simulink model "wheel_robot"  (R2019b)
settings: Solver=ode4  StartTime=0.0  StopTime=33  FixedStep=1e-2  RelTol=1e-3
values from neighbouring files (symbols this model uses):
  dt = 1e-2    (= 0.01)    [init.m]
  g = [0 0 -10]    [init.m]
  gps_pos_local_rsm = 1.66    [init.m]
  gps_vel_local_rsm = 0.05    [init.m]
  imu_acc_rsm = 0.25    [init.m]
  imu_rot_vel_rsm = 0.05    [init.m]
  initial_ctrl = [0;0]    [init.m]
  initial_state_local = [0;0;0]    [init.m]
  sqrtP0 = chol(P0,'lower')    [init.m]
  sqrtQ = chol(Q,'lower')    [init.m]
  sqrtR = chol(R,'lower')    [init.m]
  X0 = [0 0 0    0 0 0    0 0 0]'    [init.m]
libraries: simulink x1
settings Model: Creator=shawinmihail  LastModifiedBy=shawinmihail

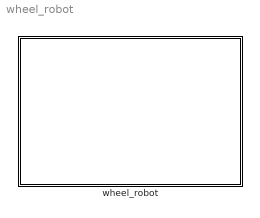
== system wheel_robot ==
  wheel_robot : Subsystem  InitFcn=init

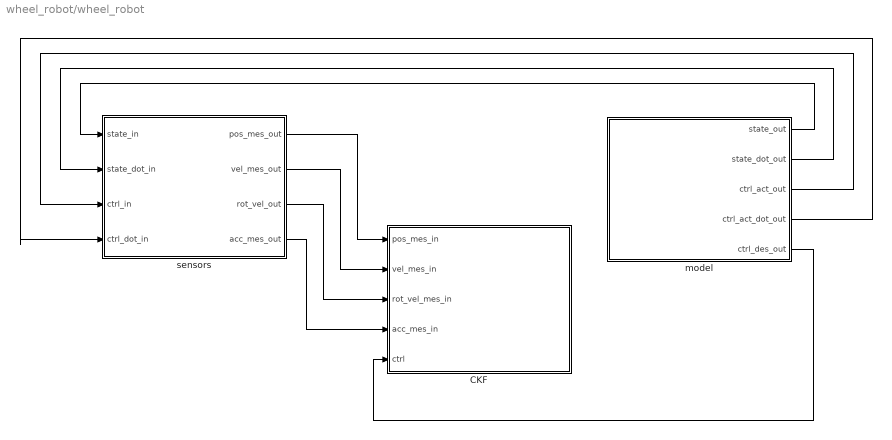
== system wheel_robot/wheel_robot ==
  CKF : Subsystem  InitFcn=init
  model : Subsystem
  sensors : Subsystem  InitFcn=init
  wires:
  model/2(state_dot_out) -> sensors/2(state_dot_in)
  model/1(state_out) -> sensors/1(state_in)
  model/3(ctrl_act_out) -> sensors/3(ctrl_in)
  model/4(ctrl_act_dot_out) -> sensors/4(ctrl_dot_in)
  sensors/4(acc_mes_out) -> CKF/4(acc_mes_in)
  sensors/3(rot_vel_out) -> CKF/3(rot_vel_mes_in)
  sensors/2(vel_mes_out) -> CKF/2(vel_mes_in)
  sensors/1(pos_mes_out) -> CKF/1(pos_mes_in)
  model/5(ctrl_des_out) -> CKF/5(ctrl)

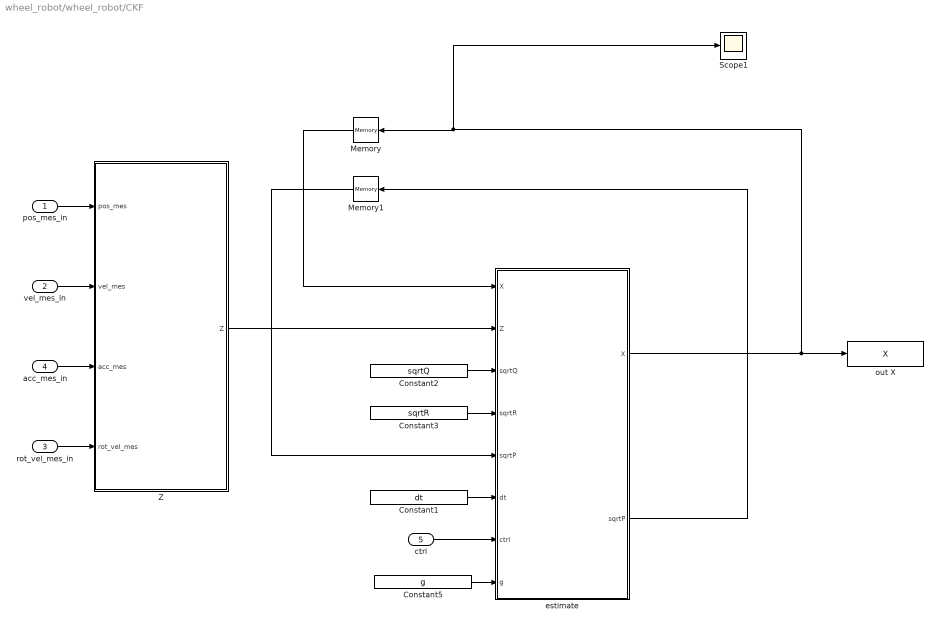
== system wheel_robot/wheel_robot/CKF ==
  pos_mes_in : Inport
  vel_mes_in : Inport  Port=2
  rot_vel_mes_in : Inport  Port=3
  acc_mes_in : Inport  Port=4
  ctrl : Inport  Port=5
  Constant1 : Constant  Value=dt
  Constant2 : Constant  Value=sqrtQ
  Constant3 : Constant  Value=sqrtR
  Constant5 : Constant  Value=g
  Memory : Memory  InitialCondition=X0
  Memory1 : Memory  InitialCondition=sqrtP0
  Scope1 : Scope
  Z : MATLAB Function  TreatAsAtomicUnit=on
  estimate : MATLAB Function  TreatAsAtomicUnit=on
  out X : ToWorkspace  VariableName=X  SaveFormat=Timeseries  SampleTime=-1
  wires:
  pos_mes_in/1 -> Z/1(pos_mes)
  vel_mes_in/1 -> Z/2(vel_mes)
  acc_mes_in/1 -> Z/3(acc_mes)
  rot_vel_mes_in/1 -> Z/4(rot_vel_mes)
  Z/1(Z) -> estimate/2(Z)
  ctrl/1 -> estimate/7(ctrl)
  estimate/1(X) -> Memory/1, Scope1/1, out X/1
  Memory/1 -> estimate/1("X ")
  Constant5/1 -> estimate/8(g)
  Constant1/1 -> estimate/6(dt)
  Memory1/1 -> estimate/5("sqrtP ")
  Constant2/1 -> estimate/3(sqrtQ)
  Constant3/1 -> estimate/4(sqrtR)
  estimate/2(sqrtP) -> Memory1/1

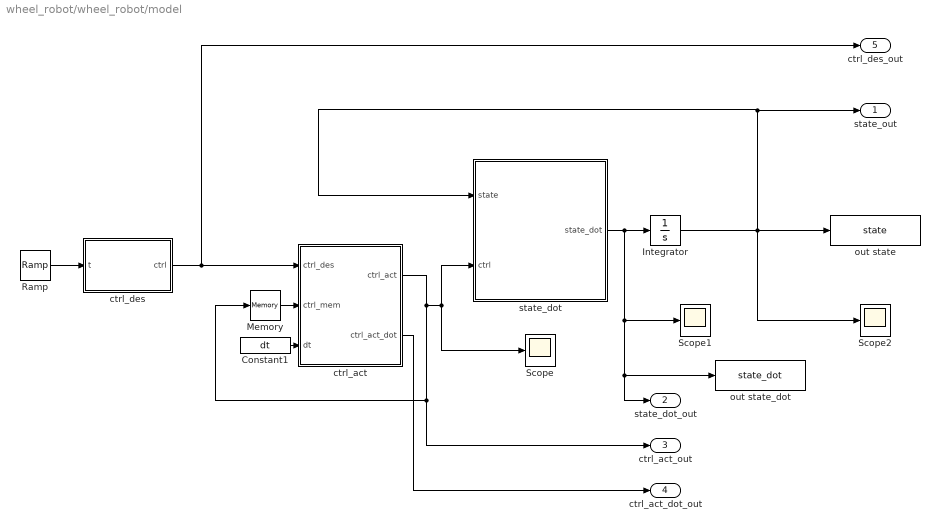
== system wheel_robot/wheel_robot/model ==
  Constant1 : Constant  Value=dt
  Integrator : Integrator  InitialCondition=initial_state_local
  Memory : Memory  InitialCondition=initial_ctrl
  Ramp : simulink/Sources/Ramp  slope=1  start=0  InitialOutput=0
  Scope : Scope
  Scope1 : Scope
  Scope2 : Scope
  ctrl_act : MATLAB Function  TreatAsAtomicUnit=on
  ctrl_des : MATLAB Function  TreatAsAtomicUnit=on
  out state : ToWorkspace  VariableName=state  SaveFormat=Timeseries  SampleTime=-1
  out state_dot : ToWorkspace  VariableName=state_dot  SaveFormat=Timeseries  SampleTime=-1
  state_dot : MATLAB Function  TreatAsAtomicUnit=on
  state_out : Outport
  state_dot_out : Outport  Port=2
  ctrl_act_out : Outport  Port=3
  ctrl_act_dot_out : Outport  Port=4
  ctrl_des_out : Outport  Port=5
  wires:
  state_dot/1(state_dot) -> out state_dot/1, state_dot_out/1, Scope1/1, Integrator/1
  Integrator/1 -> state_dot/1(state), state_out/1, out state/1, Scope2/1
  Ramp/1 -> ctrl_des/1(t)
  ctrl_des/1(ctrl) -> ctrl_des_out/1, ctrl_act/1(ctrl_des)
  ctrl_act/1(ctrl_act) -> ctrl_act_out/1, Memory/1, state_dot/2(ctrl), Scope/1
  Memory/1 -> ctrl_act/2(ctrl_mem)
  Constant1/1 -> ctrl_act/3(dt)
  ctrl_act/2(ctrl_act_dot) -> ctrl_act_dot_out/1

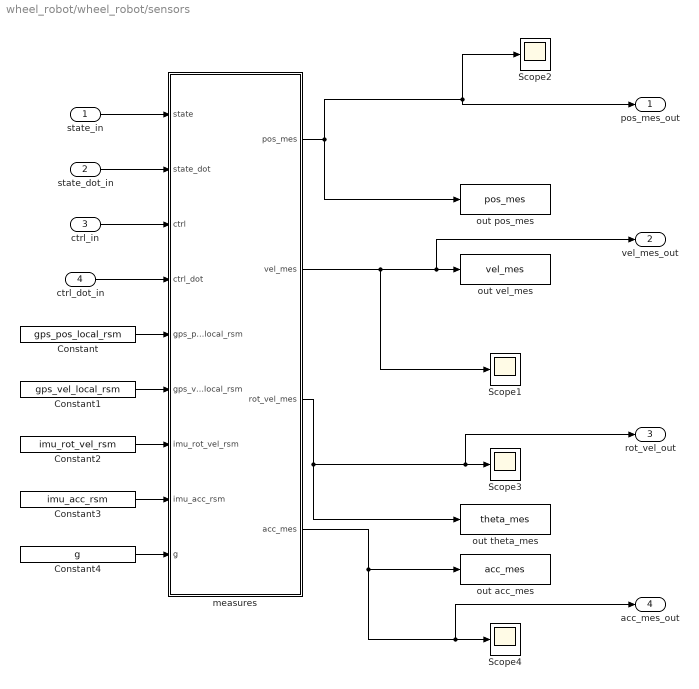
== system wheel_robot/wheel_robot/sensors ==
  state_in : Inport
  state_dot_in : Inport  Port=2
  ctrl_in : Inport  Port=3
  ctrl_dot_in : Inport  Port=4
  Constant : Constant  Value=gps_pos_local_rsm
  Constant1 : Constant  Value=gps_vel_local_rsm
  Constant2 : Constant  Value=imu_rot_vel_rsm
  Constant3 : Constant  Value=imu_acc_rsm
  Constant4 : Constant  Value=g
  Scope{1..4} (4 alike) : Scope
  measures : MATLAB Function  TreatAsAtomicUnit=on
  out acc_mes : ToWorkspace  VariableName=acc_mes  SaveFormat=Timeseries  SampleTime=-1
  out pos_mes : ToWorkspace  VariableName=pos_mes  SaveFormat=Timeseries  SampleTime=-1
  out theta_mes : ToWorkspace  VariableName=theta_mes  SaveFormat=Timeseries  SampleTime=-1
  out vel_mes : ToWorkspace  VariableName=vel_mes  SaveFormat=Timeseries  SampleTime=-1
  pos_mes_out : Outport
  vel_mes_out : Outport  Port=2
  rot_vel_out : Outport  Port=3
  acc_mes_out : Outport  Port=4
  wires:
  state_in/1 -> measures/1(state)
  state_dot_in/1 -> measures/2(state_dot)
  measures/2(vel_mes) -> Scope1/1, vel_mes_out/1, out vel_mes/1
  measures/1(pos_mes) -> pos_mes_out/1, Scope2/1, out pos_mes/1
  measures/3(rot_vel_mes) -> out theta_mes/1, rot_vel_out/1, Scope3/1
  Constant/1 -> measures/5(gps_pos_local_rsm)
  Constant1/1 -> measures/6(gps_vel_local_rsm)
  Constant2/1 -> measures/7(imu_rot_vel_rsm)
  ctrl_in/1 -> measures/3(ctrl)
  ctrl_dot_in/1 -> measures/4(ctrl_dot)
  measures/4(acc_mes) -> acc_mes_out/1, Scope4/1, out acc_mes/1
  Constant3/1 -> measures/8(imu_acc_rsm)
  Constant4/1 -> measures/9(g)

== matlab function wheel_robot/model/ctrl_des ==
  data: t input; ctrl output
function ctrl = fcn(t)
ctrl = [0.5; 0.3*(cos(t/2))];

== matlab function wheel_robot/model/state_dot ==
  data: state input; state_dot output; ctrl input
function state_dot = fcn(state, ctrl)
% state = [x; y; theta]
% ctrl = [u; v]

x = state(1);
y = state(2);
theta = state(3);

v = ctrl(1);
u = ctrl(2);

x_dot = v*cos(theta);
y_dot = v*sin(theta);
theta_dot = v*u;

state_dot = [x_dot; y_dot; theta_dot];

== matlab function wheel_robot/model/ctrl_act ==
  data: ctrl_des input; ctrl_act output; ctrl_mem input; dt input; ctrl_act_dot output
function [ctrl_act, ctrl_act_dot] = fcn(ctrl_des, ctrl_mem, dt)
p_v = 1;
p_u = 0.5;
ctrl_act_dot = [p_v * (ctrl_des(1) - ctrl_mem(1)); p_u * (ctrl_des(2) - ctrl_mem(2))];
ctrl_act = ctrl_mem + ctrl_act_dot*dt;

== matlab function wheel_robot/CKF/Z ==
  settings: updateMethod=DISCRETE
  data: pos_mes input; Z output; vel_mes input; acc_mes input; rot_vel_mes input
function Z  = fcn(pos_mes, vel_mes, acc_mes, rot_vel_mes)

% Z = [r v a w]

Z = [pos_mes; vel_mes; acc_mes; rot_vel_mes];

== matlab function wheel_robot/sensors/measures ==
  settings: updateMethod=DISCRETE
  data: state input; pos_mes output; state_dot input; ctrl input; ctrl_dot input; vel_mes output; rot_vel_mes output; gps_pos_local_rsm input; gps_vel_local_rsm input; imu_rot_vel_rsm input; imu_acc_rsm input; acc_mes output; g input
function [pos_mes, vel_mes, rot_vel_mes, acc_mes] = fcn(state, state_dot, ctrl, ctrl_dot, gps_pos_local_rsm, gps_vel_local_rsm, imu_rot_vel_rsm, imu_acc_rsm, g)

x = state(1);
y = state(2);
theta = state(3);

x_dot = state_dot(1);
y_dot = state_dot(2);
theta_dot = state_dot(3);

v = ctrl(1);
u = ctrl(2);

v_dot = ctrl_dot(1);
u_dot = ctrl_dot(2);

pos_mes_noise = gps_pos_local_rsm * randn(3,1);
pos_mes = [x; y; 0] + pos_mes_noise;

vel_mes_noise = gps_vel_local_rsm * randn(3,1);
vel_mes = [x_dot; y_dot; 0] + vel_mes_noise;

rot_vel_noise = imu_rot_vel_rsm * randn(3,1);
rot_vel_mes = [0; 0; theta] + rot_vel_noise;

acc_noise = imu_acc_rsm * randn(3,1);
acc_mes = [v_dot; 0; 0] + g + acc_noise; %% pitch and roll is zero now

== matlab function wheel_robot/CKF/estimate ==
  settings: updateMethod=DISCRETE
  data: X input; Z input; sqrtQ input; sqrtR input; sqrtP input; dt input; ctrl input; X output; g input; sqrtP output
function [X, sqrtP]  = fcn(X, Z, sqrtQ, sqrtR, sqrtP,  dt, ctrl, g)

% X = [r v eul(ZYX)]
% Z = [r v a w]

[X, sqrtP] = wheel_robot_ckf(X, Z, sqrtQ, sqrtR, sqrtP,  dt, ctrl, g);
